simulink model "jerkControl2017"  (Simulink 8.9)
settings: Solver=FixedStepDiscrete  StartTime=0.0  StopTime="Config.SIMULATION_TIME "  FixedStep=Config.Ts  RelTol=1e-3  EnableMultiTasking=on
InitFcn:
  | %% initialize the simulation
  | cd(fileparts(which(bdroot)));
  | initJerkControl;
StopFcn:
  | %% stop the simulation
  | cd(fileparts(which(bdroot)));
  | stopJerkControl;
undefined symbols (not defined in the file or in its folder): Config, DiscIntNeverNeededParam, Gain, Reg, ROBOT_DOF, Sat, Sm
libraries: WBToolboxLibrary x69, simulink x4
(part 1 of 2)
settings Model: Creator=daniele  LastModifiedBy=gnava
settings DataIOCC: SignalLoggingSaveFormat=Dataset
settings OptimizationCC: ExpressionDepthLimit=2147483647  ZeroExternalMemoryAtStartup=off
settings DebuggingCC: SolverPrmCheckMsg=warning  AllowSymbolicDim=off
settings SFSimCC: SimParseCustomCode=off
settings RTWCC: GenCodeOnly=on  TargetLang=C++
settings GRTTargetCC: TargetLangStandard=C++03 (ISO)  CombineOutputUpdateFcns=on  MatFileLogging=off  CodeInterfacePackaging=C++ class  SupportNonFinite=off  GRTInterface=off
settings CPPComponent: GenerateDestructor=on  GenerateExternalIOAccessMethods=None  ParameterMemberVisibility=private  InternalMemberVisibility=private  GenerateParameterAccessMethods=None  GenerateInternalMemberAccessMethods=None  UseOperatorNewForModelRefRegistration=off

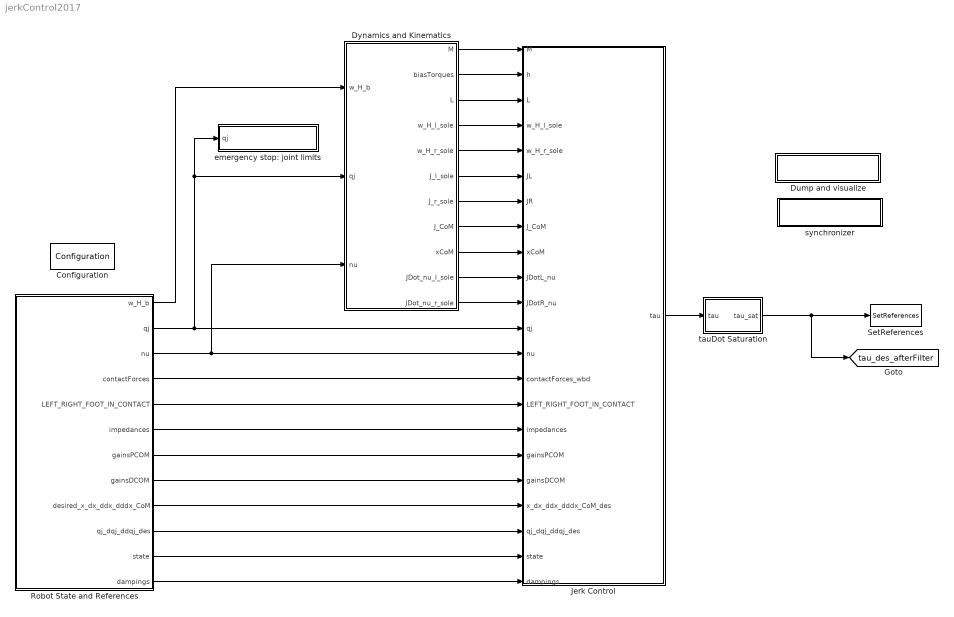
== system jerkControl2017 ==
  Configuration : WBToolboxLibrary/Utilities/Configuration  ConfigSource=Workspace  ConfigObject='WBTConfigRobot'  RobotName='icubSim'  UrdfFile='model.urdf'  ControlledJoints={'l_elbow','l_shoulder_pitch','torso_roll'}  ControlBoardsNames={'left_arm','right_arm','torso'}  LocalName='WBT'  GravityVector=[0,0,-9.81]
      settings: SourceProductName=WholeBodyToolbox
  Dump and visualize : Subsystem
      mask Display: disp('VISUALIZER')
  Dynamics and Kinematics : Subsystem
  Jerk Control : Subsystem
  Robot State and References : Subsystem  Priority=-10
  SetReferences : WBToolboxLibrary/Actuators/SetReferences  controlType=Torque  refSpeed=50  refAcceleration=1000000*(pi/180)
      settings: SourceProductName=WholeBodyToolbox
  emergency stop: joint limits : Subsystem
      mask Display: disp('EMERGENCY STOP')
  synchronizer : Subsystem
      mask Display: disp('SYNCHRONIZER')
  tauDot Saturation : Subsystem
  tag scope: tau_des_afterFilter=global
  wires:
  tauDot Saturation/1(tau_sat) -> SetReferences/1, [tau_des_afterFilter]
  Dynamics and Kinematics/1(M) -> Jerk Control/1(M)
  Dynamics and Kinematics/2(biasTorques) -> Jerk Control/2(h)
  Dynamics and Kinematics/3(L) -> Jerk Control/3(L)
  Dynamics and Kinematics/4(w_H_l_sole) -> Jerk Control/4(w_H_l_sole)
  Dynamics and Kinematics/5(w_H_r_sole) -> Jerk Control/5(w_H_r_sole)
  Dynamics and Kinematics/6(J_l_sole) -> Jerk Control/6(JL)
  Dynamics and Kinematics/7(J_r_sole) -> Jerk Control/7(JR)
  Dynamics and Kinematics/8(J_CoM) -> Jerk Control/8(J_CoM)
  Dynamics and Kinematics/9(xCoM) -> Jerk Control/9(xCoM)
  Dynamics and Kinematics/10(JDot_nu_l_sole) -> Jerk Control/10(JDotL_nu)
  Dynamics and Kinematics/11(JDot_nu_r_sole) -> Jerk Control/11(JDotR_nu)
  Robot State and References/1(w_H_b) -> Dynamics and Kinematics/1(w_H_b)
  Robot State and References/2(qj) -> Jerk Control/12(qj), emergency stop: joint limits/1(qj), Dynamics and Kinematics/2(qj)
  Robot State and References/3(nu) -> Jerk Control/13(nu), Dynamics and Kinematics/3(nu)
  Robot State and References/5(LEFT_RIGHT_FOOT_IN_CONTACT) -> Jerk Control/15(LEFT_RIGHT_FOOT_IN_CONTACT)
  Robot State and References/6(impedances) -> Jerk Control/16(impedances)
  Robot State and References/7(gainsPCOM) -> Jerk Control/17(gainsPCOM)
  Robot State and References/8(gainsDCOM) -> Jerk Control/18(gainsDCOM)
  Robot State and References/9(desired_x_dx_ddx_dddx_CoM) -> Jerk Control/19(x_dx_ddx_dddx_CoM_des)
  Robot State and References/10(qj_dqj_ddqj_des) -> Jerk Control/20(qj_dqj_ddqj_des)
  Jerk Control/1("tau ") -> tauDot Saturation/1(tau)
  Robot State and References/4(contactForces) -> Jerk Control/14(contactForces_wbd)
  Robot State and References/11(state) -> Jerk Control/21(state)
  Robot State and References/12(dampings) -> Jerk Control/22(dampings)

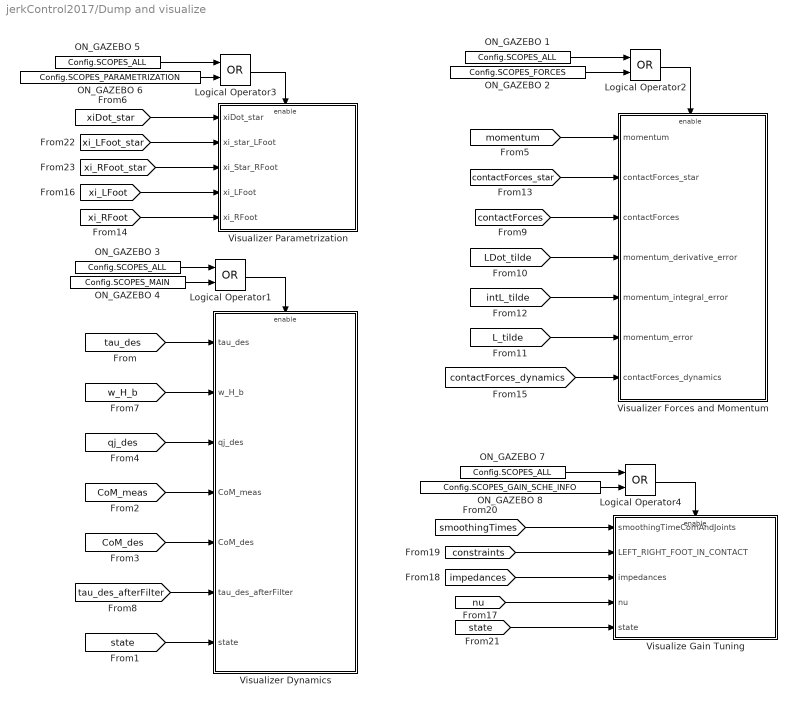
== system jerkControl2017/Dump and visualize ==
  Logical Operator{1..4} (4 alike) : Logic  Operator=OR  AllPortsSameDT=off  OutDataTypeStr=boolean
  ON_GAZEBO {1,3,5,7} (4 alike) : Constant  Value=Config.SCOPES_ALL
  ON_GAZEBO 2 : Constant  Value=Config.SCOPES_FORCES
  ON_GAZEBO 4 : Constant  Value=Config.SCOPES_MAIN
  ON_GAZEBO 6 : Constant  Value=Config.SCOPES_PARAMETRIZATION
  ON_GAZEBO 8 : Constant  Value=Config.SCOPES_GAIN_SCHE_INFO
  "Visualize Gain Tuning  " : Subsystem
  Visualizer Dynamics : Subsystem
  Visualizer Forces and Momentum : Subsystem
  Visualizer Parametrization : Subsystem
  wires:
  ON_GAZEBO 3/1 -> Logical Operator1/1
  ON_GAZEBO 4/1 -> Logical Operator1/2
  Logical Operator1/1 -> Visualizer Dynamics/Enable
  [state] -> Visualizer Dynamics/7(state)
  [CoM_meas] -> Visualizer Dynamics/4(CoM_meas)
  [qj_des] -> Visualizer Dynamics/3(qj_des)
  [w_H_b] -> Visualizer Dynamics/2(w_H_b)
  [tau_des] -> Visualizer Dynamics/1(tau_des)
  [CoM_des] -> Visualizer Dynamics/5(CoM_des)
  [tau_des_afterFilter] -> Visualizer Dynamics/6(tau_des_afterFilter)
  Logical Operator2/1 -> Visualizer Forces and Momentum/Enable
  ON_GAZEBO 2/1 -> Logical Operator2/2
  ON_GAZEBO 1/1 -> Logical Operator2/1
  [momentum] -> Visualizer Forces and Momentum/1(momentum)
  [xiDot_star] -> Visualizer Parametrization/1(xiDot_star)
  ON_GAZEBO 5/1 -> Logical Operator3/1
  Logical Operator3/1 -> Visualizer Parametrization/Enable
  ON_GAZEBO 6/1 -> Logical Operator3/2
  [contactForces_star] -> Visualizer Forces and Momentum/2(contactForces_star)
  [contactForces] -> Visualizer Forces and Momentum/3(contactForces)
  [LDot_tilde] -> Visualizer Forces and Momentum/4(momentum_derivative_error)
  [intL_tilde] -> Visualizer Forces and Momentum/5(momentum_integral_error)
  [L_tilde] -> Visualizer Forces and Momentum/6(momentum_error)
  [contactForces_dynamics] -> Visualizer Forces and Momentum/7(contactForces_dynamics)
  ON_GAZEBO 7/1 -> Logical Operator4/1
  ON_GAZEBO 8/1 -> Logical Operator4/2
  Logical Operator4/1 -> "Visualize Gain Tuning  "/Enable
  [nu] -> "Visualize Gain Tuning  "/4(nu)
  [impedances] -> "Visualize Gain Tuning  "/3(impedances)
  [constraints] -> "Visualize Gain Tuning  "/2(LEFT_RIGHT_FOOT_IN_CONTACT)
  [smoothingTimes] -> "Visualize Gain Tuning  "/1(smoothingTimeComAndJoints)
  [state] -> "Visualize Gain Tuning  "/5(state)
  [xi_LFoot_star] -> Visualizer Parametrization/2(xi_star_LFoot)
  [xi_RFoot] -> Visualizer Parametrization/5(xi_RFoot)
  [xi_LFoot] -> Visualizer Parametrization/4(xi_LFoot)
  [xi_RFoot_star] -> Visualizer Parametrization/3(xi_Star_RFoot)

== system jerkControl2017/Dynamics and Kinematics ==
  w_H_b : Inport
  qj : Inport  Port=2
  nu : Inport  Port=3
  Dynamics : Subsystem
  Kinematics : Subsystem
  M : Outport
  biasTorques : Outport  Port=2
  L : Outport  Port=3
  w_H_l_sole : Outport  Port=4
  w_H_r_sole : Outport  Port=5
  J_l_sole : Outport  Port=6
  J_r_sole : Outport  Port=7
  J_CoM : Outport  Port=8
  xCoM : Outport  Port=9
  JDot_nu_l_sole : Outport  Port=10
  JDot_nu_r_sole : Outport  Port=11
  wires:
  w_H_b/1 -> Kinematics/3(w_H_b), Dynamics/1(w_H_b)
  qj/1 -> Dynamics/2(qj), Kinematics/2(qj)
  nu/1 -> Dynamics/3(nu), Kinematics/1(nu)
  Dynamics/1(M) -> M/1
  Dynamics/2(biasTorques) -> biasTorques/1
  Dynamics/3(L) -> L/1
  Kinematics/7(JDot_nu_l_sole) -> JDot_nu_l_sole/1
  Kinematics/8(JDot_nu_r_sole) -> JDot_nu_r_sole/1
  Kinematics/4(J_r_sole) -> J_r_sole/1
  Kinematics/1(w_H_l_sole) -> w_H_l_sole/1
  Kinematics/3(J_l_sole) -> J_l_sole/1
  Kinematics/5(J_CoM) -> J_CoM/1
  Kinematics/6(xCoM) -> xCoM/1
  Kinematics/2(w_H_r_sole) -> w_H_r_sole/1

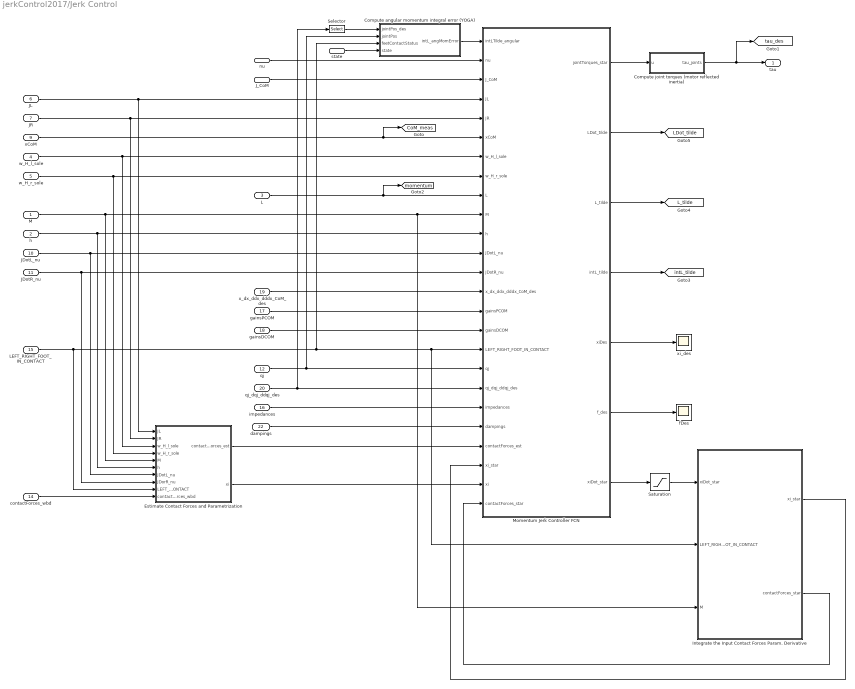
== system jerkControl2017/Jerk Control ==
  M : Inport
  h : Inport  Port=2
  L : Inport  Port=3
  w_H_l_sole : Inport  Port=4
  w_H_r_sole : Inport  Port=5
  JL : Inport  Port=6
  JR : Inport  Port=7
  J_CoM : Inport  Port=8
  xCoM : Inport  Port=9
  JDotL_nu : Inport  Port=10
  JDotR_nu : Inport  Port=11
  qj : Inport  Port=12
  nu : Inport  Port=13
  contactForces_wbd : Inport  Port=14
  LEFT_RIGHT_FOOT_IN_CONTACT : Inport  Port=15
  impedances : Inport  Port=16
  gainsPCOM : Inport  Port=17
  gainsDCOM : Inport  Port=18
  x_dx_ddx_dddx_CoM_des : Inport  Port=19
  qj_dqj_ddqj_des : Inport  Port=20
  state : Inport  Port=21
  dampings : Inport  Port=22
  Compute angular momentum integral error (YOGA) : Subsystem
  Compute joint torques (motor reflected inertia) : Subsystem
  Estimate Contact Forces and Parametrization : Subsystem
  Integrate the Input Contact Forces Param. Derivative : Subsystem
  "Momentum Jerk Controller FCN " : MATLAB Function  TreatAsAtomicUnit=on
  Saturation : Saturate  UpperLimit=Sat.xiDot  LowerLimit=-Sat.xiDot
  Selector : Selector  NumberOfDimensions=2  InputPortWidth=3  IndexOptions=Index vector (dialog),Index vector (dialog)  Indices=[1:ROBOT_DOF],1  OutputSizes=1,1
  fDes : Scope
  xi_des : Scope
  "tau " : Outport
  tag scope: CoM_meas=global, LDot_tilde=global, L_tilde=global, intL_tilde=global, momentum=global, tau_des=global
  wires:
  w_H_l_sole/1 -> Estimate Contact Forces and Parametrization/3(w_H_l_sole), "Momentum Jerk Controller FCN "/7(w_H_l_sole)
  w_H_r_sole/1 -> "Momentum Jerk Controller FCN "/8(w_H_r_sole), Estimate Contact Forces and Parametrization/4(w_H_r_sole)
  x_dx_ddx_dddx_CoM_des/1 -> "Momentum Jerk Controller FCN "/14(x_dx_ddx_dddx_CoM_des)
  nu/1 -> "Momentum Jerk Controller FCN "/2(nu)
  gainsPCOM/1 -> "Momentum Jerk Controller FCN "/15(gainsPCOM)
  Compute angular momentum integral error (YOGA)/1(intL_angMomError) -> "Momentum Jerk Controller FCN "/1(intLTilde_angular)
  qj_dqj_ddqj_des/1 -> "Momentum Jerk Controller FCN "/19(qj_dqj_ddqj_des), Selector/1
  gainsDCOM/1 -> "Momentum Jerk Controller FCN "/16(gainsDCOM)
  impedances/1 -> "Momentum Jerk Controller FCN "/20(impedances)
  xCoM/1 -> "Momentum Jerk Controller FCN "/6(xCoM), [CoM_meas]
  qj/1 -> "Momentum Jerk Controller FCN "/18(qj), Compute angular momentum integral error (YOGA)/2(jointPos)
  Selector/1 -> Compute angular momentum integral error (YOGA)/1(jointPos_des)
  J_CoM/1 -> "Momentum Jerk Controller FCN "/3(J_CoM)
  "Momentum Jerk Controller FCN "/7(xiDot_star) -> Saturation/1
  h/1 -> "Momentum Jerk Controller FCN "/11(h), Estimate Contact Forces and Parametrization/6(h)
  JR/1 -> "Momentum Jerk Controller FCN "/5(JR), Estimate Contact Forces and Parametrization/2(JR)
  L/1 -> [momentum], "Momentum Jerk Controller FCN "/9(L)
  state/1 -> Compute angular momentum integral error (YOGA)/4(state)
  LEFT_RIGHT_FOOT_IN_CONTACT/1 -> Integrate the Input Contact Forces Param. Derivative/2(LEFT_RIGHT_FOOT_IN_CONTACT), "Momentum Jerk Controller FCN "/17(LEFT_RIGHT_FOOT_IN_CONTACT), Compute angular momentum integral error (YOGA)/3(feetContactStatus), Estimate Contact Forces and Parametrization/9(LEFT_RIGHT_FOOT_IN_CONTACT)
  JDotR_nu/1 -> "Momentum Jerk Controller FCN "/13(JDotR_nu), Estimate Contact Forces and Parametrization/8(JDorR_nu)
  Integrate the Input Contact Forces Param. Derivative/1(xi_star) -> "Momentum Jerk Controller FCN "/23(xi_star)
  Integrate the Input Contact Forces Param. Derivative/2(contactForces_star) -> "Momentum Jerk Controller FCN "/25(contactForces_star)
  "Momentum Jerk Controller FCN "/4(intL_tilde) -> [intL_tilde]
  "Momentum Jerk Controller FCN "/3(L_tilde) -> [L_tilde]
  "Momentum Jerk Controller FCN "/2(LDot_tilde) -> [LDot_tilde]
  dampings/1 -> "Momentum Jerk Controller FCN "/21(dampings)
  Saturation/1 -> Integrate the Input Contact Forces Param. Derivative/1(xiDot_star)
  contactForces_wbd/1 -> Estimate Contact Forces and Parametrization/10(contactForces_wbd)
  JL/1 -> "Momentum Jerk Controller FCN "/4(JL), Estimate Contact Forces and Parametrization/1(JL)
  JDotL_nu/1 -> "Momentum Jerk Controller FCN "/12(JDotL_nu), Estimate Contact Forces and Parametrization/7(JDotL_nu)
  Estimate Contact Forces and Parametrization/1(contactForces_est) -> "Momentum Jerk Controller FCN "/22(contactForces_est)
  "Momentum Jerk Controller FCN "/1(jointTorques_star) -> Compute joint torques (motor reflected inertia)/1(u)
  Compute joint torques (motor reflected inertia)/1(tau_joints) -> [tau_des], "tau "/1
  M/1 -> Integrate the Input Contact Forces Param. Derivative/3(M), "Momentum Jerk Controller FCN "/10(M), Estimate Contact Forces and Parametrization/5(M)
  Estimate Contact Forces and Parametrization/2(xi) -> "Momentum Jerk Controller FCN "/24(xi)
  "Momentum Jerk Controller FCN "/5(xiDes) -> xi_des/1
  "Momentum Jerk Controller FCN "/6(f_des) -> fDes/1

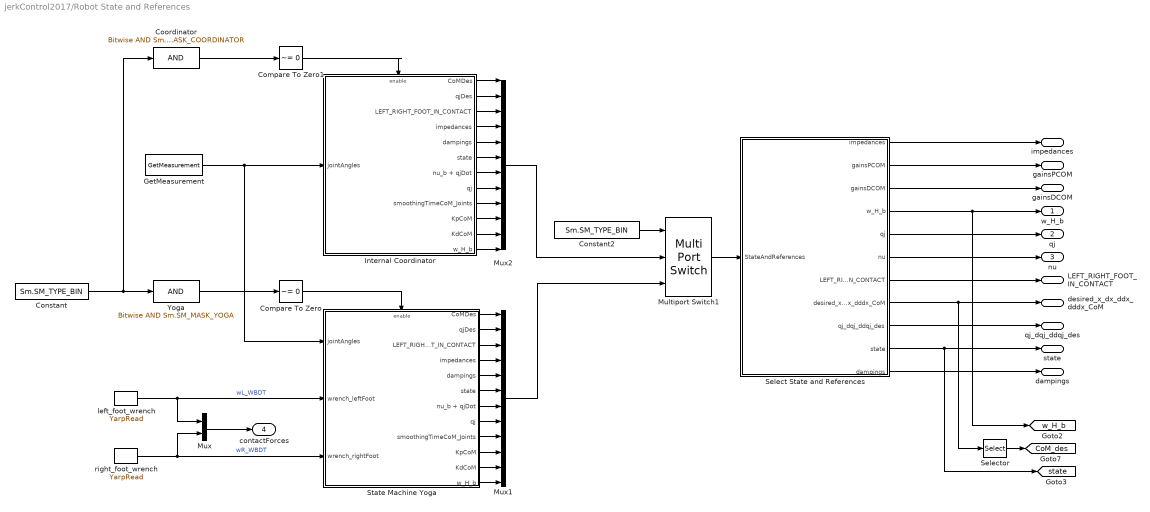
== system jerkControl2017/Robot State and References ==
  Compare To Zero : simulink/Logic and Bit Operations/Compare To Zero  relop=~=  OutDataTypeStr=boolean
  Compare To Zero1 : simulink/Logic and Bit Operations/Compare To Zero  relop=~=  OutDataTypeStr=boolean
  Constant : Constant  Priority=-10  Value=Sm.SM_TYPE_BIN  OutDataTypeStr=uint8
  Constant2 : Constant  Priority=-10  Value=Sm.SM_TYPE_BIN  OutDataTypeStr=uint8
  Coordinator : simulink/Logic and Bit Operations/Bitwise Operator  logicop=AND  UseBitMask=on  BitMask=Sm.SM_MASK_COORDINATOR  BitMaskRealWorld=Stored Integer
  GetMeasurement : WBToolboxLibrary/States/GetMeasurement  measuredType=Joints Position
      settings: SourceProductName=WholeBodyToolbox
  Internal Coordinator : Subsystem
  Multiport Switch1 : MultiPortSwitch  DataPortOrder=Specify indices  DataPortIndices={1, 2}
  Mux : Mux  Inputs=2
  Mux1 : Mux  Inputs=12
  Mux2 : Mux  Inputs=12
  Select State and References : Subsystem
  Selector : Selector  NumberOfDimensions=2  InputPortWidth=3  IndexOptions=Index vector (dialog),Index vector (dialog)  Indices=[1 2 3],[1]  OutputSizes=1,1
  State Machine Yoga : Subsystem  Priority=-100
  Yoga : simulink/Logic and Bit Operations/Bitwise Operator  logicop=AND  UseBitMask=on  BitMask=Sm.SM_MASK_YOGA  BitMaskRealWorld=Stored Integer
  left_foot_wrench : WBToolboxLibrary/Utilities/YarpRead  portName=Ports.WRENCH_LEFT_FOOT  signalSize=6  timeout=0.5  blocking=off  timestamp=off  autoconnect=on  errorOnConnection=on
      settings: SourceProductName=WholeBodyToolbox
  right_foot_wrench : WBToolboxLibrary/Utilities/YarpRead  portName=Ports.WRENCH_RIGHT_FOOT  signalSize=6  timeout=0.5  blocking=off  timestamp=off  autoconnect=on  errorOnConnection=on
      settings: SourceProductName=WholeBodyToolbox
  w_H_b : Outport
  qj : Outport  Port=2
  nu : Outport  Port=3
  contactForces : Outport  Port=4
  LEFT_RIGHT_FOOT_IN_CONTACT : Outport  Port=5
  impedances : Outport  Port=6
  gainsPCOM : Outport  Port=7
  gainsDCOM : Outport  Port=8
  desired_x_dx_ddx_dddx_CoM : Outport  Port=9
  qj_dqj_ddqj_des : Outport  Port=10
  state : Outport  Port=11
  dampings : Outport  Port=12
  tag scope: CoM_des=global, state=global, w_H_b=global
  wires:
  Constant/1 -> Coordinator/1, Yoga/1
  State Machine Yoga/3(LEFT_RIGHT_FOOT_IN_CONTACT) -> Mux1/3
  State Machine Yoga/2(qjDes) -> Mux1/2
  State Machine Yoga/1(CoMDes) -> Mux1/1
  Internal Coordinator/1(CoMDes) -> Mux2/1
  Internal Coordinator/2(qjDes) -> Mux2/2
  Internal Coordinator/3(LEFT_RIGHT_FOOT_IN_CONTACT) -> Mux2/3
  State Machine Yoga/4(impedances) -> Mux1/4
  Internal Coordinator/4(impedances) -> Mux2/4
  State Machine Yoga/6(state) -> Mux1/6
  Internal Coordinator/6(state) -> Mux2/6
  Internal Coordinator/7(nu_b + qjDot) -> Mux2/7
  Internal Coordinator/8(qj) -> Mux2/8
  State Machine Yoga/7(nu_b + qjDot) -> Mux1/7
  State Machine Yoga/8(qj) -> Mux1/8
  Coordinator/1 -> Compare To Zero1/1
  Yoga/1 -> Compare To Zero/1
  Compare To Zero/1 -> State Machine Yoga/Enable
  Compare To Zero1/1 -> Internal Coordinator/Enable
  Internal Coordinator/9(smoothingTimeCoM_Joints) -> Mux2/9
  State Machine Yoga/9(smoothingTimeCoM_Joints) -> Mux1/9
  State Machine Yoga/10(KpCoM) -> Mux1/10
  State Machine Yoga/11(KdCoM) -> Mux1/11
  Internal Coordinator/10(KpCoM) -> Mux2/10
  Internal Coordinator/11(KdCoM) -> Mux2/11
  Constant2/1 -> Multiport Switch1/1
  GetMeasurement/1 -> Internal Coordinator/1(jointAngles), State Machine Yoga/1(jointAngles)
  State Machine Yoga/12(w_H_b) -> Mux1/12
  Internal Coordinator/12(w_H_b) -> Mux2/12
  Mux2/1 -> Multiport Switch1/2
  Mux1/1 -> Multiport Switch1/3
  Multiport Switch1/1 -> Select State and References/1(StateAndReferences)
  Select State and References/1(impedances) -> impedances/1
  Select State and References/2(gainsPCOM) -> gainsPCOM/1
  Select State and References/3(gainsDCOM) -> gainsDCOM/1
  Select State and References/4(w_H_b) -> w_H_b/1, [w_H_b]
  Select State and References/5(qj) -> qj/1
  Select State and References/6(nu) -> nu/1
  Select State and References/7(LEFT_RIGHT_FOOT_IN_CONTACT) -> LEFT_RIGHT_FOOT_IN_CONTACT/1
  Select State and References/8(desired_x_dx_ddx_dddx_CoM) -> desired_x_dx_ddx_dddx_CoM/1, Selector/1
  Select State and References/9(qj_dqj_ddqj_des) -> qj_dqj_ddqj_des/1
  Select State and References/10(state) -> state/1, [state]
  Selector/1 -> [CoM_des]
  left_foot_wrench/1 -> Mux/1, State Machine Yoga/2(wrench_leftFoot)  "wL_WBDT"
  right_foot_wrench/1 -> Mux/2, State Machine Yoga/3(wrench_rightFoot)  "wR_WBDT"
  Mux/1 -> contactForces/1
  State Machine Yoga/5(dampings) -> Mux1/5
  Internal Coordinator/5(dampings) -> Mux2/5
  Select State and References/11(dampings) -> dampings/1

== system jerkControl2017/emergency stop: joint limits ==
  qj : Inport
  ON_GAZEBO 1 : Constant  Value=Config.EMERGENCY_STOP_WITH_JOINTS_LIMITS
  ON_GAZEBO 2 : Constant  Value=Config.EMERGENCY_STOP_WITH_ENCODER_SPIKES
  STOP IF JOINTS HIT THE LIMITS : Subsystem
  STOP IF THERE ARE SPIKES IN THE ENCODERS : Subsystem
  wires:
  ON_GAZEBO 1/1 -> STOP IF JOINTS HIT THE LIMITS/Enable
  qj/1 -> STOP IF THERE ARE SPIKES IN THE ENCODERS/1(qj), STOP IF JOINTS HIT THE LIMITS/1(qj)
  ON_GAZEBO 2/1 -> STOP IF THERE ARE SPIKES IN THE ENCODERS/Enable

== system jerkControl2017/synchronizer ==
  GAZEBO_SYNCHRONIZER : Subsystem
  Logical Operator : Logic  Operator=NOT  AllPortsSameDT=off  OutDataTypeStr=boolean
  "ON_GAZEBO " : Constant  Value=Config.ON_GAZEBO
  REAL_TIME_SYNC : Subsystem
  To Workspace : ToWorkspace  VariableName=yarp_time  SaveFormat=Structure With Time  SampleTime=-1
  Yarp Clock : WBToolboxLibrary/Utilities/Yarp Clock
      settings: SourceProductName=WholeBodyToolbox
  wires:
  Logical Operator/1 -> REAL_TIME_SYNC/Enable
  "ON_GAZEBO "/1 -> GAZEBO_SYNCHRONIZER/Enable, Logical Operator/1
  Yarp Clock/1 -> To Workspace/1

== system jerkControl2017/tauDot Saturation ==
  tau : Inport
  Constant : Constant  Value=Config.SATURATE_TORQUE_DERIVATIVE
  Constant1 : Constant  Value=Config.Ts
  Constant2 : Constant  Value=Sat.uDotMax
  Saturate Torque Derivative : MATLAB Function  TreatAsAtomicUnit=on
  Saturation : Saturate  UpperLimit=Sat.torque  LowerLimit=-Sat.torque
  Switch : Switch  Criteria=u2 > Threshold
  "holder " : WBToolboxLibrary/Utilities/holder 
      settings: SourceProductName=WholeBodyToolbox
  tau_sat : Outport
  wires:
  Switch/1 -> Saturation/1
  Constant/1 -> Switch/2
  Constant1/1 -> Saturate Torque Derivative/3(tStep)
  Saturate Torque Derivative/1(uSat) -> Switch/1
  "holder "/1 -> Saturate Torque Derivative/2(u_0)
  Saturation/1 -> tau_sat/1
  tau/1 -> Switch/3, Saturate Torque Derivative/1(u), "holder "/1
  Constant2/1 -> Saturate Torque Derivative/4(uDotMax)

== system jerkControl2017/Dump and visualize/Visualize Gain Tuning   ==
  smoothingTimeComAndJoints : Inport
  LEFT_RIGHT_FOOT_IN_CONTACT : Inport  Port=2
  impedances : Inport  Port=3
  nu : Inport  Port=4
  state : Inport  Port=5
  Enable : EnablePort
  Demux : Demux  Outputs=2
  Demux1 : Demux  Outputs=Config.numOfJointsForEachControlboard
  Demux2 : Demux  Outputs=Config.numOfJointsForEachControlboard
  Gain : Gain  Gain=180/pi
  Gain1 : Gain  Gain=180/pi
  Impedances : Scope  NumInputPorts=6
  Left right foot in contact : Scope
  Selector1 : Selector  InputPortWidth=6+ROBOT_DOF  IndexOptions=Index vector (dialog)  Indices=[7:6+ROBOT_DOF]  OutputSizes=1
  Selector2 : Selector  InputPortWidth=6+ROBOT_DOF  IndexOptions=Index vector (dialog)  Indices=[1:6]  OutputSizes=1
  "joint velocities " : Scope  NumInputPorts=6
  jointsSmoothingTime : Scope  NumInputPorts=2
  linear and angular  base velocity : Scope  NumInputPorts=3
  wires:
  state/1 -> "joint velocities "/6, linear and angular  base velocity/3, Impedances/6, jointsSmoothingTime/2  "state"
  LEFT_RIGHT_FOOT_IN_CONTACT/1 -> Left right foot in contact/1
  impedances/1 -> Demux1/1
  smoothingTimeComAndJoints/1 -> jointsSmoothingTime/1  "smoothingTimeComAndJoints"
  Demux1/4 -> Impedances/4  "left_leg"
  Demux1/5 -> Impedances/5  "right_leg"
  Demux1/3 -> Impedances/3  "right_arm"
  Demux1/1 -> Impedances/1  "torso"
  Demux1/2 -> Impedances/2  "left_arm"
  Selector1/1 -> Gain/1
  Demux2/4 -> "joint velocities "/4  "left_leg"
  Demux2/3 -> "joint velocities "/3  "right_arm"
  Demux2/1 -> "joint velocities "/1  "torso"
  Demux2/2 -> "joint velocities "/2  "left_arm"
  nu/1 -> Selector1/1, Selector2/1
  Selector2/1 -> Demux/1
  Demux/1 -> linear and angular  base velocity/1
  Demux/2 -> Gain1/1
  Gain/1 -> Demux2/1
  Gain1/1 -> linear and angular  base velocity/2
  Demux2/5 -> "joint velocities "/5  "right_leg"

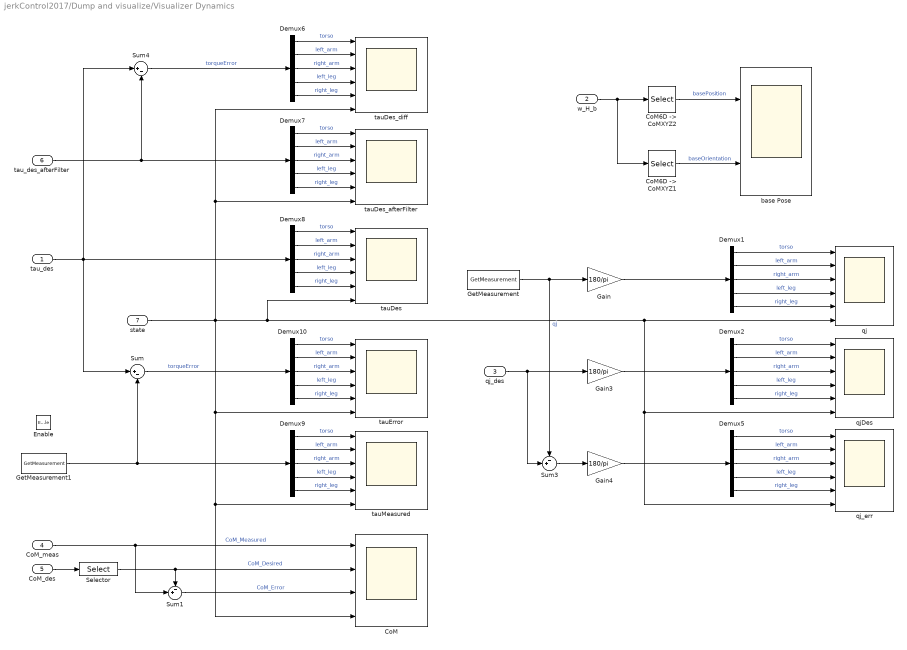
== system jerkControl2017/Dump and visualize/Visualizer Dynamics ==
  tau_des : Inport
  w_H_b : Inport  Port=2
  qj_des : Inport  Port=3
  CoM_meas : Inport  Port=4
  CoM_des : Inport  Port=5
  tau_des_afterFilter : Inport  Port=6
  state : Inport  Port=7
  Enable : EnablePort
  CoM : Scope  NumInputPorts=4
  "CoM6D ->  CoMXYZ1" : Selector  NumberOfDimensions=2  InputPortWidth=7  IndexOptions=Index vector (dialog),Index vector (dialog)  Indices=[1 2 3],[1 2 3]  OutputSizes=1,1
  "CoM6D ->  CoMXYZ2" : Selector  NumberOfDimensions=2  InputPortWidth=7  IndexOptions=Index vector (dialog),Index vector (dialog)  Indices=[1 2 3],[4]  OutputSizes=1,1
  Demux{1..2,5..10} (8 alike) : Demux  Outputs=Config.numOfJointsForEachControlboard
  Gain : Gain  Gain=180/pi
  Gain3 : Gain  Gain=180/pi
  Gain4 : Gain  Gain=180/pi
  GetMeasurement : WBToolboxLibrary/States/GetMeasurement  measuredType=Joints Position
      settings: SourceProductName=WholeBodyToolbox
  GetMeasurement1 : WBToolboxLibrary/States/GetMeasurement  measuredType=Joints Torque
      settings: SourceProductName=WholeBodyToolbox
  Selector : Selector  NumberOfDimensions=2  IndexOptions=Index vector (dialog),Index vector (dialog)  Indices=[1:3],1  OutputSizes=1,1
  Sum : Sum  Inputs=|+-
  Sum1 : Sum  Inputs=-+|
  Sum3 : Sum  Inputs=-+|
  Sum4 : Sum  Inputs=|+-
  base Pose : Scope  NumInputPorts=2
  qj : Scope  NumInputPorts=6
  qjDes : Scope  NumInputPorts=6
  qj_err : Scope  NumInputPorts=6
  tauDes : Scope  NumInputPorts=6
  tauDes_afterFilter : Scope  NumInputPorts=6
  tauDes_diff : Scope  NumInputPorts=6
  tauError : Scope  NumInputPorts=6
  tauMeasured : Scope  NumInputPorts=6
  wires:
  CoM_meas/1 -> Sum1/2, CoM/1  "CoM_Measured"
  CoM_des/1 -> Selector/1
  Gain/1 -> Demux1/1
  GetMeasurement/1 -> Gain/1, Sum3/1  "qj"
  Demux1/5 -> qj/5  "right_leg"
  Demux1/1 -> qj/1  "torso"
  Demux1/2 -> qj/2  "left_arm"
  Demux1/4 -> qj/4  "left_leg"
  Demux1/3 -> qj/3  "right_arm"
  GetMeasurement1/1 -> Demux9/1, Sum/2
  Demux8/5 -> tauDes/5  "right_leg"
  Demux8/1 -> tauDes/1  "torso"
  Demux8/2 -> tauDes/2  "left_arm"
  Demux8/4 -> tauDes/4  "left_leg"
  Demux8/3 -> tauDes/3  "right_arm"
  Demux10/5 -> tauError/5  "right_leg"
  Demux10/1 -> tauError/1  "torso"
  Demux10/2 -> tauError/2  "left_arm"
  Demux10/4 -> tauError/4  "left_leg"
  Demux10/3 -> tauError/3  "right_arm"
  Sum/1 -> Demux10/1  "torqueError"
  Demux9/5 -> tauMeasured/5  "right_leg"
  Demux9/1 -> tauMeasured/1  "torso"
  Demux9/2 -> tauMeasured/2  "left_arm"
  Demux9/4 -> tauMeasured/4  "left_leg"
  Demux9/3 -> tauMeasured/3  "right_arm"
  qj_des/1 -> Sum3/2, Gain3/1
  Gain3/1 -> Demux2/1
  Demux2/5 -> qjDes/5  "right_leg"
  Demux2/1 -> qjDes/1  "torso"
  Demux2/2 -> qjDes/2  "left_arm"
  Demux2/4 -> qjDes/4  "left_leg"
  Demux2/3 -> qjDes/3  "right_arm"
  Gain4/1 -> Demux5/1
  Demux5/5 -> qj_err/5  "right_leg"
  Demux5/1 -> qj_err/1  "torso"
  Demux5/2 -> qj_err/2  "left_arm"
  Demux5/4 -> qj_err/4  "left_leg"
  Demux5/3 -> qj_err/3  "right_arm"
  Sum3/1 -> Gain4/1
  Selector/1 -> Sum1/1, CoM/2  "CoM_Desired"
  w_H_b/1 -> "CoM6D ->  CoMXYZ1"/1, "CoM6D ->  CoMXYZ2"/1
  "CoM6D ->  CoMXYZ2"/1 -> base Pose/1  "basePosition"
  "CoM6D ->  CoMXYZ1"/1 -> base Pose/2  "baseOrientation"
  Demux7/4 -> tauDes_afterFilter/4  "left_leg"
  Demux7/5 -> tauDes_afterFilter/5  "right_leg"
  Demux7/2 -> tauDes_afterFilter/2  "left_arm"
  Demux7/1 -> tauDes_afterFilter/1  "torso"
  Demux7/3 -> tauDes_afterFilter/3  "right_arm"
  tau_des_afterFilter/1 -> Demux7/1, Sum4/2
  Sum4/1 -> Demux6/1  "torqueError"
  tau_des/1 -> Demux8/1, Sum/1, Sum4/1
  Demux6/5 -> tauDes_diff/5  "right_leg"
  state/1 -> tauDes_diff/6, tauDes_afterFilter/6, qj_err/6, qjDes/6, qj/6, tauDes/6, CoM/4, tauMeasured/6, tauError/6
  Demux6/3 -> tauDes_diff/3  "right_arm"
  Demux6/2 -> tauDes_diff/2  "left_arm"
  Demux6/4 -> tauDes_diff/4  "left_leg"
  Demux6/1 -> tauDes_diff/1  "torso"
  Sum1/1 -> CoM/3  "CoM_Error"

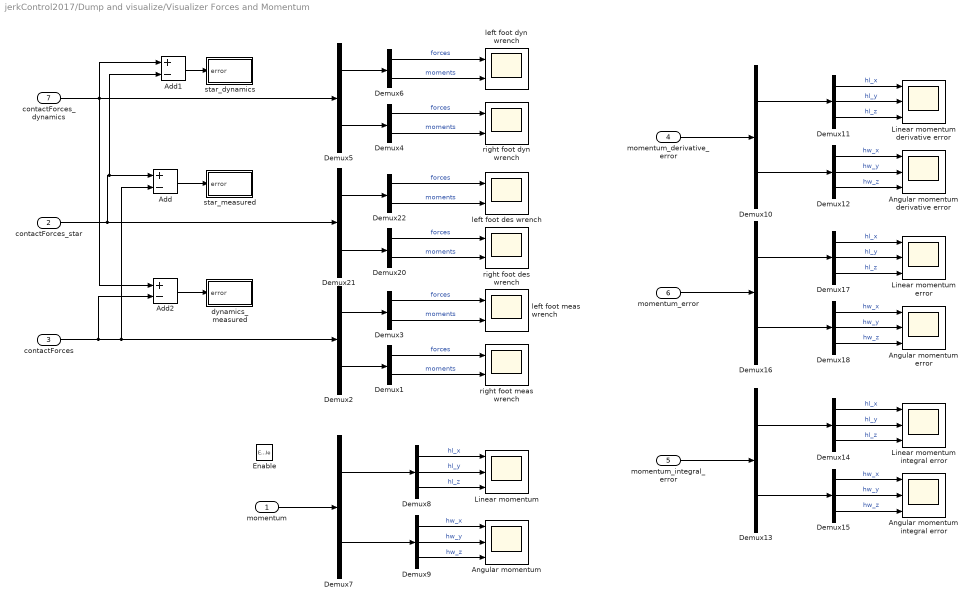
== system jerkControl2017/Dump and visualize/Visualizer Forces and Momentum ==
  momentum : Inport
  contactForces_star : Inport  Port=2
  contactForces : Inport  Port=3
  momentum_derivative_error : Inport  Port=4
  momentum_integral_error : Inport  Port=5
  momentum_error : Inport  Port=6
  contactForces_dynamics : Inport  Port=7
  Enable : EnablePort
  Add : Sum  Inputs=+-
  Add1 : Sum  Inputs=+-
  Add2 : Sum  Inputs=+-
  Angular momentum : Scope  NumInputPorts=3
  Angular momentum derivative error : Scope  NumInputPorts=3
  Angular momentum error : Scope  NumInputPorts=3
  Angular momentum integral error : Scope  NumInputPorts=3
  Demux{1,3..4,6,20,22} (6 alike) : Demux  Outputs=[3;3]
  Demux{7,10,13,16} (4 alike) : Demux  Outputs=2
  Demux{8..9,11..12,14..15,17..18} (8 alike) : Demux  Outputs=3
  Demux2 : Demux  Outputs=[6;6]
  Demux21 : Demux  Outputs=[6;6]
  Demux5 : Demux  Outputs=[6;6]
  Linear momentum : Scope  NumInputPorts=3
  Linear momentum derivative error : Scope  NumInputPorts=3
  Linear momentum error : Scope  NumInputPorts=3
  Linear momentum integral error : Scope  NumInputPorts=3
  dynamics_measured : Subsystem
  left foot des wrench : Scope  NumInputPorts=2
  left foot dyn wrench : Scope  NumInputPorts=2
  left foot meas wrench : Scope  NumInputPorts=2
  right foot des wrench : Scope  NumInputPorts=2
  right foot dyn wrench : Scope  NumInputPorts=2
  right foot meas wrench : Scope  NumInputPorts=2
  star_dynamics : Subsystem
  star_measured : Subsystem
  wires:
  Demux9/3 -> Angular momentum/3  "hw_z"
  Demux8/1 -> Linear momentum/1  "hl_x"
  Demux8/2 -> Linear momentum/2  "hl_y"
  Demux7/2 -> Demux9/1
  Demux9/2 -> Angular momentum/2  "hw_y"
  Demux7/1 -> Demux8/1
  momentum/1 -> Demux7/1
  Demux8/3 -> Linear momentum/3  "hl_z"
  Demux9/1 -> Angular momentum/1  "hw_x"
  Demux11/1 -> Linear momentum derivative error/1  "hl_x"
  momentum_derivative_error/1 -> Demux10/1
  Demux10/1 -> Demux11/1
  Demux12/1 -> Angular momentum derivative error/1  "hw_x"
  Demux12/2 -> Angular momentum derivative error/2  "hw_y"
  Demux11/2 -> Linear momentum derivative error/2  "hl_y"
  Demux11/3 -> Linear momentum derivative error/3  "hl_z"
  Demux10/2 -> Demux12/1
  Demux12/3 -> Angular momentum derivative error/3  "hw_z"
  Demux14/1 -> Linear momentum integral error/1  "hl_x"
  momentum_integral_error/1 -> Demux13/1
  Demux13/1 -> Demux14/1
  Demux15/1 -> Angular momentum integral error/1  "hw_x"
  Demux15/2 -> Angular momentum integral error/2  "hw_y"
  Demux14/2 -> Linear momentum integral error/2  "hl_y"
  Demux14/3 -> Linear momentum integral error/3  "hl_z"
  Demux13/2 -> Demux15/1
  Demux15/3 -> Angular momentum integral error/3  "hw_z"
  Demux17/1 -> Linear momentum error/1  "hl_x"
  momentum_error/1 -> Demux16/1
  Demux16/1 -> Demux17/1
  Demux18/1 -> Angular momentum error/1  "hw_x"
  Demux18/2 -> Angular momentum error/2  "hw_y"
  Demux17/2 -> Linear momentum error/2  "hl_y"
  Demux17/3 -> Linear momentum error/3  "hl_z"
  Demux16/2 -> Demux18/1
  Demux18/3 -> Angular momentum error/3  "hw_z"
  Demux20/2 -> right foot des wrench/2  "moments"
  Demux21/2 -> Demux20/1
  Demux21/1 -> Demux22/1
  Demux22/2 -> left foot des wrench/2  "moments"
  Demux22/1 -> left foot des wrench/1  "forces"
  Demux20/1 -> right foot des wrench/1  "forces"
  Demux3/2 -> left foot meas wrench/2  "moments"
  Demux3/1 -> left foot meas wrench/1  "forces"
  Demux1/2 -> right foot meas wrench/2  "moments"
  Demux1/1 -> right foot meas wrench/1  "forces"
  Demux2/1 -> Demux3/1
  Demux2/2 -> Demux1/1
  Demux4/2 -> right foot dyn wrench/2  "moments"
  Demux6/2 -> left foot dyn wrench/2  "moments"
  Demux6/1 -> left foot dyn wrench/1  "forces"
  Demux5/2 -> Demux4/1
  Demux4/1 -> right foot dyn wrench/1  "forces"
  Demux5/1 -> Demux6/1
  Add/1 -> star_measured/1(error)
  contactForces_star/1 -> Add1/2, Add/1, Demux21/1
  Add1/1 -> star_dynamics/1(error)
  contactForces_dynamics/1 -> Add2/1, Demux5/1, Add1/1
  contactForces/1 -> Add2/2, Add/2, Demux2/1
  Add2/1 -> dynamics_measured/1(error)

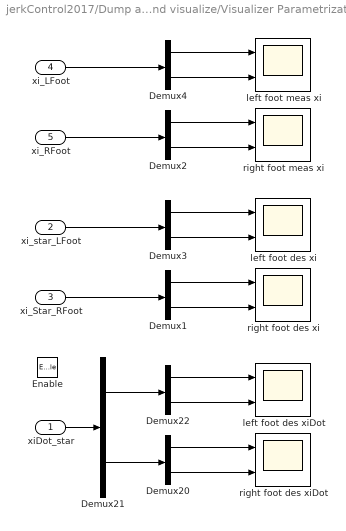
== system jerkControl2017/Dump and visualize/Visualizer Parametrization ==
  xiDot_star : Inport
  xi_star_LFoot : Inport  Port=2
  xi_Star_RFoot : Inport  Port=3
  xi_LFoot : Inport  Port=4
  xi_RFoot : Inport  Port=5
  Enable : EnablePort
  Demux{1..4,20,22} (6 alike) : Demux  Outputs=[3;3]
  Demux21 : Demux  Outputs=[6;6]
  left foot des xi : Scope  NumInputPorts=2
  left foot des xiDot : Scope  NumInputPorts=2
  left foot meas xi : Scope  NumInputPorts=2
  right foot des xi : Scope  NumInputPorts=2
  right foot des xiDot : Scope  NumInputPorts=2
  right foot meas xi : Scope  NumInputPorts=2
  wires:
  Demux20/1 -> right foot des xiDot/1
  Demux21/1 -> Demux22/1
  Demux22/2 -> left foot des xiDot/2
  Demux21/2 -> Demux20/1
  xiDot_star/1 -> Demux21/1
  Demux22/1 -> left foot des xiDot/1
  Demux20/2 -> right foot des xiDot/2
  Demux3/2 -> left foot des xi/2
  xi_star_LFoot/1 -> Demux3/1
  Demux3/1 -> left foot des xi/1
  xi_Star_RFoot/1 -> Demux1/1
  Demux1/1 -> right foot des xi/1
  Demux1/2 -> right foot des xi/2
  Demux2/2 -> right foot meas xi/2
  Demux4/2 -> left foot meas xi/2
  xi_RFoot/1 -> Demux2/1
  Demux2/1 -> right foot meas xi/1
  xi_LFoot/1 -> Demux4/1
  Demux4/1 -> left foot meas xi/1

== system jerkControl2017/Dynamics and Kinematics/Dynamics ==
  w_H_b : Inport
  qj : Inport  Port=2
  nu : Inport  Port=3
  Add motors reflected inertia : Subsystem
  CentroidalMomentum : WBToolboxLibrary/Model/Dynamics/CentroidalMomentum
      settings: SourceProductName=WholeBodyToolbox
  "CoM6D ->  CoMXYZ1" : Selector  InputPortWidth=6+ROBOT_DOF  IndexOptions=Index vector (dialog)  Indices=[7:6+ROBOT_DOF]  OutputSizes=1
  "CoM6D ->  CoMXYZ2" : Selector  InputPortWidth=6+ROBOT_DOF  IndexOptions=Index vector (dialog)  Indices=[1 2 3 4 5 6]  OutputSizes=1
  GetBiasForces : WBToolboxLibrary/Model/Dynamics/GetBiasForces
      settings: SourceProductName=WholeBodyToolbox
  MassMatrix : WBToolboxLibrary/Model/Dynamics/MassMatrix
      settings: SourceProductName=WholeBodyToolbox
  M : Outport
  biasTorques : Outport  Port=2
  L : Outport  Port=3
  wires:
  CentroidalMomentum/1 -> L/1
  GetBiasForces/1 -> biasTorques/1
  w_H_b/1 -> CentroidalMomentum/1, GetBiasForces/1, MassMatrix/1
  qj/1 -> CentroidalMomentum/2, GetBiasForces/2, MassMatrix/2
  "CoM6D ->  CoMXYZ1"/1 -> CentroidalMomentum/4, GetBiasForces/4
  nu/1 -> "CoM6D ->  CoMXYZ1"/1, "CoM6D ->  CoMXYZ2"/1
  MassMatrix/1 -> Add motors reflected inertia/1(M)
  Add motors reflected inertia/1(M_with_motor_inertia) -> M/1
  "CoM6D ->  CoMXYZ2"/1 -> CentroidalMomentum/3, GetBiasForces/3

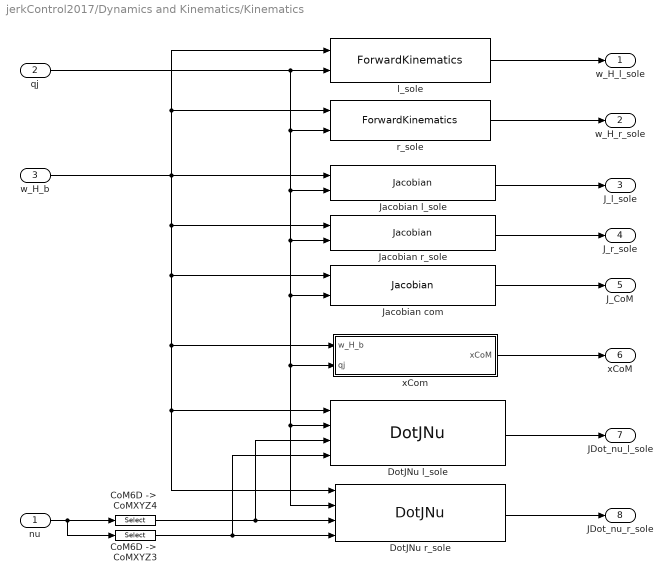
== system jerkControl2017/Dynamics and Kinematics/Kinematics ==
  nu : Inport
  qj : Inport  Port=2
  w_H_b : Inport  Port=3
  "CoM6D ->  CoMXYZ3" : Selector  InputPortWidth=6+ROBOT_DOF  IndexOptions=Index vector (dialog)  Indices=[7:6+ROBOT_DOF]  OutputSizes=1
  "CoM6D ->  CoMXYZ4" : Selector  InputPortWidth=6+ROBOT_DOF  IndexOptions=Index vector (dialog)  Indices=[1 2 3 4 5 6]  OutputSizes=1
  "DotJNu l_sole " : WBToolboxLibrary/Model/Jacobians/DotJNu  frameName=Frames.LEFT_FOOT
      settings: SourceProductName=WholeBodyToolbox
  "DotJNu r_sole   " : WBToolboxLibrary/Model/Jacobians/DotJNu  frameName=Frames.RIGHT_FOOT
      settings: SourceProductName=WholeBodyToolbox
  Jacobian com : WBToolboxLibrary/Model/Jacobians/Jacobian  frameName=Frames.COM
      settings: SourceProductName=WholeBodyToolbox
  Jacobian l_sole : WBToolboxLibrary/Model/Jacobians/Jacobian  frameName=Frames.LEFT_FOOT
      settings: SourceProductName=WholeBodyToolbox
  Jacobian r_sole : WBToolboxLibrary/Model/Jacobians/Jacobian  frameName=Frames.RIGHT_FOOT
      settings: SourceProductName=WholeBodyToolbox
  l_sole : WBToolboxLibrary/Model/Kinematics/ForwardKinematics  frameName=Frames.LEFT_FOOT
      settings: SourceProductName=WholeBodyToolbox
  r_sole : WBToolboxLibrary/Model/Kinematics/ForwardKinematics  frameName=Frames.RIGHT_FOOT
      settings: SourceProductName=WholeBodyToolbox
  xCom : Subsystem
  w_H_l_sole : Outport
  w_H_r_sole : Outport  Port=2
  J_l_sole : Outport  Port=3
  J_r_sole : Outport  Port=4
  J_CoM : Outport  Port=5
  xCoM : Outport  Port=6
  JDot_nu_l_sole : Outport  Port=7
  JDot_nu_r_sole : Outport  Port=8
  wires:
  "CoM6D ->  CoMXYZ3"/1 -> "DotJNu r_sole   "/4, "DotJNu l_sole "/4
  "CoM6D ->  CoMXYZ4"/1 -> "DotJNu r_sole   "/3, "DotJNu l_sole "/3
  nu/1 -> "CoM6D ->  CoMXYZ3"/1, "CoM6D ->  CoMXYZ4"/1
  w_H_b/1 -> Jacobian com/1, "DotJNu l_sole "/1, "DotJNu r_sole   "/1, xCom/1(w_H_b), Jacobian r_sole/1, Jacobian l_sole/1, r_sole/1, l_sole/1
  qj/1 -> Jacobian com/2, xCom/2(qj), "DotJNu r_sole   "/2, "DotJNu l_sole "/2, Jacobian r_sole/2, Jacobian l_sole/2, r_sole/2, l_sole/2
  l_sole/1 -> w_H_l_sole/1
  r_sole/1 -> w_H_r_sole/1
  Jacobian l_sole/1 -> J_l_sole/1
  Jacobian r_sole/1 -> J_r_sole/1
  Jacobian com/1 -> J_CoM/1
  xCom/1(xCoM) -> xCoM/1
  "DotJNu l_sole "/1 -> JDot_nu_l_sole/1
  "DotJNu r_sole   "/1 -> JDot_nu_r_sole/1

== system jerkControl2017/Jerk Control/Compute angular momentum integral error (YOGA) ==
  jointPos_des : Inport
  jointPos : Inport  Port=2
  feetContactStatus : Inport  Port=3
  state : Inport  Port=4
  Add : Sum  Inputs=-+
  CentroidalMomentum : WBToolboxLibrary/Model/Dynamics/CentroidalMomentum
      settings: SourceProductName=WholeBodyToolbox
  Compute base to fixed link transform : Subsystem
  Get Equivalent Base Velocity : MATLAB Function  TreatAsAtomicUnit=on
  Jacobian : WBToolboxLibrary/Model/Jacobians/Jacobian  frameName=Frames.LEFT_FOOT
      settings: SourceProductName=WholeBodyToolbox
  Jacobian1 : WBToolboxLibrary/Model/Jacobians/Jacobian  frameName=Frames.RIGHT_FOOT
      settings: SourceProductName=WholeBodyToolbox
  Select base to world transform : MATLAB Function  TreatAsAtomicUnit=on
  Selector : Selector  InputPortWidth=6  IndexOptions=Index vector (dialog)  Indices=[4 5 6]  OutputSizes=1
  Switch : Switch  Criteria=u2 > Threshold  Threshold=0.1
  intL_angMomError : Outport
  wires:
  jointPos_des/1 -> Add/1, Jacobian1/2, Jacobian/2, CentroidalMomentum/2, Compute base to fixed link transform/1(jointPos)
  jointPos/1 -> Add/2
  Add/1 -> Get Equivalent Base Velocity/4(jointPos_err), CentroidalMomentum/4
  Get Equivalent Base Velocity/1(baseVel_equivalent) -> CentroidalMomentum/3
  CentroidalMomentum/1 -> Selector/1
  Selector/1 -> intL_angMomError/1
  state/1 -> Select base to world transform/1(state)
  Select base to world transform/1(booleanState) -> Switch/2
  Switch/1 -> CentroidalMomentum/1, Jacobian/1, Jacobian1/1
  Compute base to fixed link transform/1(fixed_l_sole_H_b) -> Switch/1
  Compute base to fixed link transform/2(fixed_r_sole_H_b) -> Switch/3
  Jacobian/1 -> Get Equivalent Base Velocity/1(J_l_sole)
  Jacobian1/1 -> Get Equivalent Base Velocity/2(J_r_sole)
  feetContactStatus/1 -> Get Equivalent Base Velocity/3(feetContactStatus)

== system jerkControl2017/Jerk Control/Compute joint torques (motor reflected inertia) ==
  u : Inport
  " 2" : Constant  Value=Config.USE_MOTOR_REFLECTED_INERTIA
  " 3" : Constant  Value=Config.USE_DES_JOINT_ACC_FOR_MOTORS_INERTIA
  "(transpose(T*Gamma))^{-1}*I_m*(T*Gamma)^{-1}1" : MATLAB Function  TreatAsAtomicUnit=on
  Add1 : Sum  Inputs=-+
  Gain1 : Gain  Gain=Config.K_ff
  GetMeasurement1 : WBToolboxLibrary/States/GetMeasurement  measuredType=Joints Acceleration
      settings: SourceProductName=WholeBodyToolbox
  Product1 : Product  Multiplication=Matrix(*)
  Switch2 : Switch  Criteria=u2 > Threshold
  Switch3 : Switch  Criteria=u2 > Threshold
  tau_joints : Outport
  wires:
  " 3"/1 -> Switch3/2
  GetMeasurement1/1 -> Switch3/3
  [qjDDot_des] -> Switch3/1
  " 2"/1 -> Switch2/2
  Switch3/1 -> Product1/2
  Switch2/1 -> tau_joints/1
  Gain1/1 -> Add1/1
  Product1/1 -> Gain1/1
  "(transpose(T*Gamma))^{-1}*I_m*(T*Gamma)^{-1}1"/1(reflectedInertia) -> Product1/1
  u/1 -> Add1/2, Switch2/3
  Add1/1 -> Switch2/1

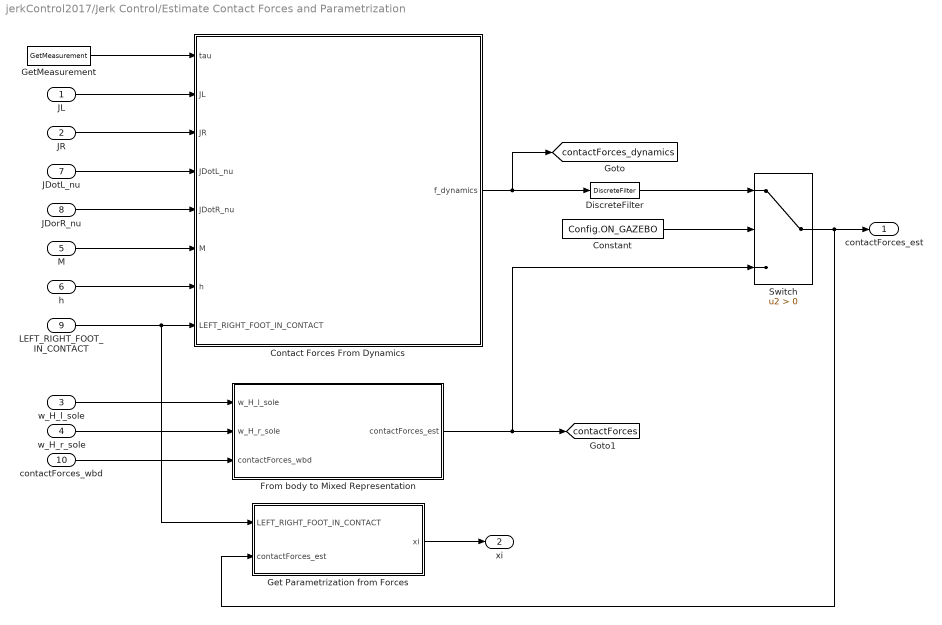
== system jerkControl2017/Jerk Control/Estimate Contact Forces and Parametrization ==
  JL : Inport
  JR : Inport  Port=2
  w_H_l_sole : Inport  Port=3
  w_H_r_sole : Inport  Port=4
  M : Inport  Port=5
  h : Inport  Port=6
  JDotL_nu : Inport  Port=7
  JDorR_nu : Inport  Port=8
  LEFT_RIGHT_FOOT_IN_CONTACT : Inport  Port=9
  contactForces_wbd : Inport  Port=10
  Constant : Constant  Value=Config.ON_GAZEBO
  Contact Forces From Dynamics : MATLAB Function  TreatAsAtomicUnit=on
  DiscreteFilter : WBToolboxLibrary/Utilities/DiscreteFilter  filterType=FirstOrderLowPassFilter  numCoeffs=[0]  denCoeffs=[0]  Fc=10  Ts=Config.Ts  orderMedianFilter=0  initStatus=on  y0=[0;0;150;0;0;0;0;0;150;0;0;0]  u0=[0]
      settings: SourceProductName=WholeBodyToolbox
  From body to Mixed Representation : Subsystem
  Get Parametrization from Forces : Subsystem
  GetMeasurement : WBToolboxLibrary/States/GetMeasurement  measuredType=Joints Torque
      settings: SourceProductName=WholeBodyToolbox
  Switch : Switch  Criteria=u2 > Threshold
  contactForces_est : Outport
  xi : Outport  Port=2
  tag scope: contactForces=global, contactForces_dynamics=global
  wires:
  JDorR_nu/1 -> Contact Forces From Dynamics/5(JDotR_nu)
  JR/1 -> Contact Forces From Dynamics/3(JR)
  JDotL_nu/1 -> Contact Forces From Dynamics/4(JDotL_nu)
  LEFT_RIGHT_FOOT_IN_CONTACT/1 -> Get Parametrization from Forces/1(LEFT_RIGHT_FOOT_IN_CONTACT), Contact Forces From Dynamics/8(LEFT_RIGHT_FOOT_IN_CONTACT)
  h/1 -> Contact Forces From Dynamics/7(h)
  M/1 -> Contact Forces From Dynamics/6(M)
  JL/1 -> Contact Forces From Dynamics/2(JL)
  contactForces_wbd/1 -> From body to Mixed Representation/3(contactForces_wbd)
  w_H_r_sole/1 -> From body to Mixed Representation/2(w_H_r_sole)
  w_H_l_sole/1 -> From body to Mixed Representation/1(w_H_l_sole)
  Switch/1 -> contactForces_est/1, Get Parametrization from Forces/2(contactForces_est)
  From body to Mixed Representation/1(contactForces_est) -> Switch/3, [contactForces]
  Contact Forces From Dynamics/1(f_dynamics) -> DiscreteFilter/1, [contactForces_dynamics]
  GetMeasurement/1 -> Contact Forces From Dynamics/1(tau)
  DiscreteFilter/1 -> Switch/1
  Get Parametrization from Forces/1(xi) -> xi/1
  Constant/1 -> Switch/2

== system jerkControl2017/Jerk Control/Integrate the Input Contact Forces Param. Derivative ==
  xiDot_star : Inport
  LEFT_RIGHT_FOOT_IN_CONTACT : Inport  Port=2
  M : Inport  Port=3
  Demux xiDot : Subsystem
  Discrete-Time Integrator3 : DiscreteIntegrator  ExternalReset=rising  InitialConditionSource=external  InitialConditionSetting=State (most efficient)  SampleTime=Config.Ts  ICPrevOutput=DiscIntNeverNeededParam  ICPrevScaledInput=DiscIntNeverNeededParam
  Discrete-Time Integrator4 : DiscreteIntegrator  ExternalReset=rising  InitialConditionSource=external  InitialConditionSetting=State (most efficient)  SampleTime=Config.Ts  ICPrevOutput=DiscIntNeverNeededParam  ICPrevScaledInput=DiscIntNeverNeededParam
  From Parametrization to Forces : Subsystem
  MatrixMultiply1 : Product
  MatrixMultiply2 : Product
  Mux : Mux  Inputs=2
  Mux1 : Mux  Inputs=2
  deadZone : Subsystem
  xi_star : Outport
  contactForces_star : Outport  Port=2
  tag scope: contactForces_star=global, xiDot_star=global, xi_LFoot_star=global, xi_RFoot_star=global
  wires:
  xiDot_star/1 -> [xiDot_star], deadZone/1(u)
  Demux xiDot/4(xiDot_RFoot) -> Discrete-Time Integrator4/1
  Demux xiDot/5(RFootContactActivation) -> MatrixMultiply2/2, From Parametrization to Forces/4(RFootContactActivation), Discrete-Time Integrator4/2
  Demux xiDot/1(xiDot_LFoot) -> Discrete-Time Integrator3/1
  Mux/1 -> [contactForces_star], contactForces_star/1
  Demux xiDot/2(LFootContactActivation) -> MatrixMultiply1/1, From Parametrization to Forces/1(LFootContactActivation), Discrete-Time Integrator3/2
  deadZone/1(u_cut) -> Demux xiDot/1(xiDot_star)
  LEFT_RIGHT_FOOT_IN_CONTACT/1 -> Demux xiDot/2(LEFT_RIGHT_FOOT_IN_CONTACT)
  M/1 -> Demux xiDot/3(M)
  Demux xiDot/6(init_xi_RFoot) -> Discrete-Time Integrator4/3
  Demux xiDot/3(init_xi_LFoot) -> Discrete-Time Integrator3/3
  Discrete-Time Integrator3/1 -> MatrixMultiply1/2, From Parametrization to Forces/2(xi_LFoot)
  Discrete-Time Integrator4/1 -> From Parametrization to Forces/3(xi_RFoot), MatrixMultiply2/1
  MatrixMultiply1/1 -> Mux1/1, [xi_LFoot_star]
  From Parametrization to Forces/1(contactForces_LFoot) -> Mux/1
  From Parametrization to Forces/2(contactForces_RFoot) -> Mux/2
  MatrixMultiply2/1 -> Mux1/2, [xi_RFoot_star]
  Mux1/1 -> xi_star/1

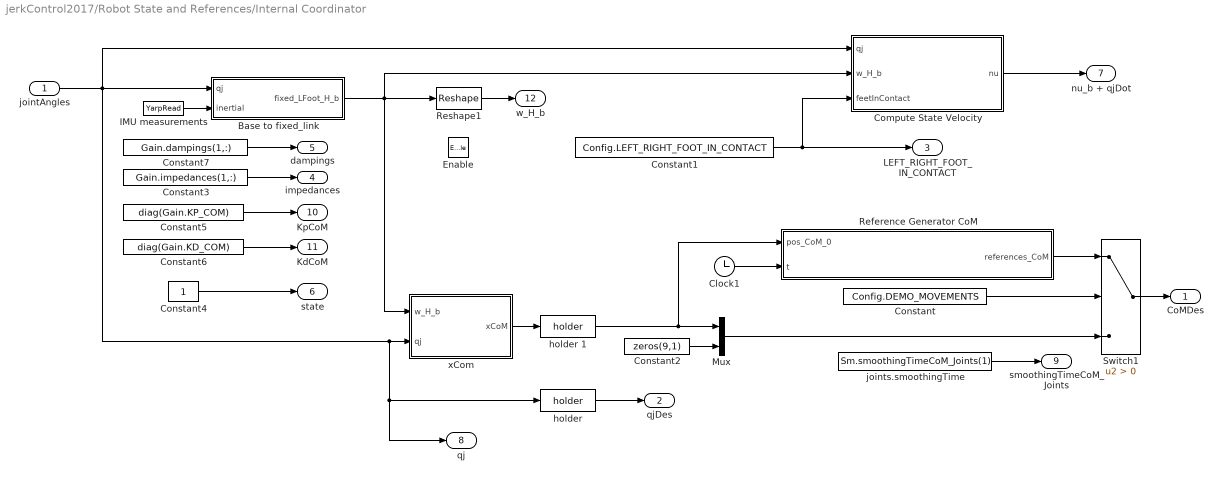
== system jerkControl2017/Robot State and References/Internal Coordinator ==
  jointAngles : Inport
  Enable : EnablePort
  Base to fixed_link : Subsystem
  Clock1 : Clock
  Compute State Velocity : Subsystem
  Constant : Constant  Value=Config.DEMO_MOVEMENTS
  Constant1 : Constant  Value=Config.LEFT_RIGHT_FOOT_IN_CONTACT
  Constant2 : Constant  Value=zeros(9,1)
  Constant3 : Constant  Value=Gain.impedances(1,:)
  Constant4 : Constant
  Constant5 : Constant  Value=diag(Gain.KP_COM)
  Constant6 : Constant  Value=diag(Gain.KD_COM)
  Constant7 : Constant  Value=Gain.dampings(1,:)
  IMU measurements : WBToolboxLibrary/Utilities/YarpRead  portName=Ports.IMU  signalSize=12  timeout=0.5  blocking=off  timestamp=off  autoconnect=on  errorOnConnection=on
      settings: SourceProductName=WholeBodyToolbox
  Mux : Mux  Inputs=2
  Reference Generator CoM : MATLAB Function  TreatAsAtomicUnit=on
  Reshape1 : Reshape  OutputDimensions=[4;4]
  Switch1 : Switch  Criteria=u2 > Threshold
  "holder " : WBToolboxLibrary/Utilities/holder 
      settings: SourceProductName=WholeBodyToolbox
  holder 1 : WBToolboxLibrary/Utilities/holder 
      settings: SourceProductName=WholeBodyToolbox
  joints.smoothingTime : Constant  Value=Sm.smoothingTimeCoM_Joints(1)
  xCom : Subsystem
  CoMDes : Outport
  qjDes : Outport  Port=2
  LEFT_RIGHT_FOOT_IN_CONTACT : Outport  Port=3
  impedances : Outport  Port=4
  dampings : Outport  Port=5
  state : Outport  Port=6
  nu_b + qjDot : Outport  Port=7
  qj : Outport  Port=8
  smoothingTimeCoM_Joints : Outport  Port=9
  KpCoM : Outport  Port=10
  KdCoM : Outport  Port=11
  w_H_b : Outport  Port=12
  wires:
  Constant/1 -> Switch1/2
  "holder "/1 -> qjDes/1
  Switch1/1 -> CoMDes/1
  Mux/1 -> Switch1/3
  Constant2/1 -> Mux/2
  Constant3/1 -> impedances/1
  Constant4/1 -> state/1
  Compute State Velocity/1(nu) -> nu_b + qjDot/1
  holder 1/1 -> Reference Generator CoM/1(pos_CoM_0), Mux/1
  xCom/1(xCoM) -> holder 1/1
  joints.smoothingTime/1 -> smoothingTimeCoM_Joints/1
  jointAngles/1 -> Compute State Velocity/1(qj), Base to fixed_link/1(qj), qj/1, "holder "/1, xCom/2(qj)
  Constant5/1 -> KpCoM/1
  Constant6/1 -> KdCoM/1
  Reshape1/1 -> w_H_b/1
  Constant1/1 -> Compute State Velocity/3("feetInContact "), LEFT_RIGHT_FOOT_IN_CONTACT/1
  IMU measurements/1 -> Base to fixed_link/2(inertial)
  Clock1/1 -> Reference Generator CoM/2(t)
  Reference Generator CoM/1(references_CoM) -> Switch1/1
  Base to fixed_link/1(fixed_LFoot_H_b) -> Compute State Velocity/2(w_H_b), xCom/1(w_H_b), Reshape1/1
  Constant7/1 -> dampings/1

== system jerkControl2017/Robot State and References/Select State and References ==
  StateAndReferences : Inport
  Compute CoM and Joint References : Subsystem
  Demux : Demux  Outputs=[12,ROBOT_DOF,2,ROBOT_DOF,ROBOT_DOF,1,ROBOT_DOF+6,ROBOT_DOF,1,3,3,16]
  Reshape1 : Reshape  OutputDimensionality=Customize  OutputDimensions=[4;4]
  impedances : Outport
  gainsPCOM : Outport  Port=2
  gainsDCOM : Outport  Port=3
  w_H_b : Outport  Port=4
  qj : Outport  Port=5
  nu : Outport  Port=6
  LEFT_RIGHT_FOOT_IN_CONTACT : Outport  Port=7
  desired_x_dx_ddx_dddx_CoM : Outport  Port=8
  qj_dqj_ddqj_des : Outport  Port=9
  state : Outport  Port=10
  dampings : Outport  Port=11
  tag scope: constraints=global, impedances=global, nu=global, smoothingTimes=global
  wires:
  Demux/8 -> qj/1  "qj"
  Demux/6 -> state/1  "state"
  Demux/9 -> [smoothingTimes], Compute CoM and Joint References/3(smoothingTimeMinJerk_CoMDes_qjDes)  "smoothingTimeMinJerk_CoMDes_qjDes"
  Demux/7 -> nu/1, [nu]  "nu"
  StateAndReferences/1 -> Demux/1
  Demux/4 -> [impedances], impedances/1  "impedances"
  Demux/3 -> [constraints], LEFT_RIGHT_FOOT_IN_CONTACT/1  "constraints"
  Reshape1/1 -> w_H_b/1
  Demux/1 -> Compute CoM and Joint References/1(CoMDes)  "CoMDes"
  Demux/2 -> Compute CoM and Joint References/2(qjDes)  "qjDes"
  Compute CoM and Joint References/1(x_dx_ddx_dddx_CoM_des) -> desired_x_dx_ddx_dddx_CoM/1
  Compute CoM and Joint References/2(qj_dqj_ddqj_des) -> qj_dqj_ddqj_des/1
  Demux/12 -> Reshape1/1
  Demux/11 -> gainsDCOM/1
  Demux/10 -> gainsPCOM/1
  Demux/5 -> dampings/1  "dampings"

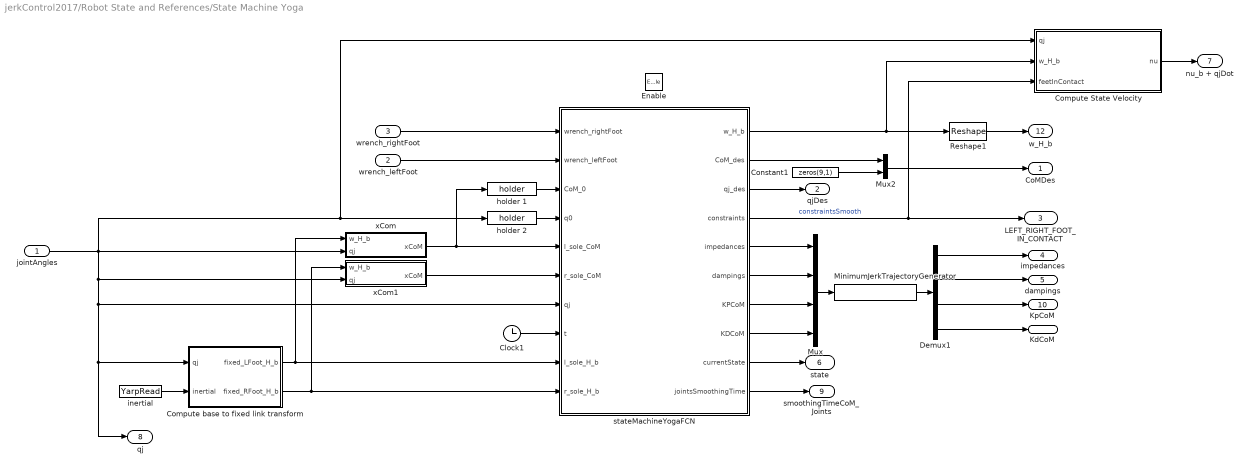
== system jerkControl2017/Robot State and References/State Machine Yoga ==
  jointAngles : Inport
  wrench_leftFoot : Inport  Port=2
  wrench_rightFoot : Inport  Port=3
  Enable : EnablePort
  Clock1 : Clock
  Compute State Velocity : Subsystem
  Compute base to fixed link transform : Subsystem
  Constant1 : Constant  Value=zeros(9,1)
  Demux1 : Demux  Outputs=[ROBOT_DOF,ROBOT_DOF,3,3]
  MinimumJerkTrajectoryGenerator : WBToolboxLibrary/Utilities/MinimumJerkTrajectoryGenerator  externalSettlingTime=off  settlingTime=Gain.SmoothingTimeGainScheduling  sampleTime=Config.Ts  resetOnSettlingTime=off  firstDerivatives=off  secondDerivatives=off  explicitInitialValue=off
      settings: SourceProductName=WholeBodyToolbox
  Mux : Mux
  Mux2 : Mux  Inputs=2
  Reshape1 : Reshape  OutputDimensions=[4;4]
  holder 1 : WBToolboxLibrary/Utilities/holder 
      settings: SourceProductName=WholeBodyToolbox
  holder 2 : WBToolboxLibrary/Utilities/holder 
      settings: SourceProductName=WholeBodyToolbox
  inertial : WBToolboxLibrary/Utilities/YarpRead  portName=Ports.IMU  signalSize=12  timeout=0.5  blocking=off  timestamp=off  autoconnect=on  errorOnConnection=off
      settings: SourceProductName=WholeBodyToolbox
  stateMachineYogaFCN : MATLAB Function  TreatAsAtomicUnit=on
  xCom : Subsystem
  xCom1 : Subsystem
  CoMDes : Outport
  qjDes : Outport  Port=2
  LEFT_RIGHT_FOOT_IN_CONTACT : Outport  Port=3
  impedances : Outport  Port=4
  dampings : Outport  Port=5
  state : Outport  Port=6
  nu_b + qjDot : Outport  Port=7
  qj : Outport  Port=8
  smoothingTimeCoM_Joints : Outport  Port=9
  KpCoM : Outport  Port=10
  KdCoM : Outport  Port=11
  w_H_b : Outport  Port=12
  wires:
  xCom/1(xCoM) -> holder 1/1, stateMachineYogaFCN/5(l_sole_CoM)
  holder 1/1 -> stateMachineYogaFCN/3(CoM_0)
  holder 2/1 -> stateMachineYogaFCN/4(q0)
  Clock1/1 -> stateMachineYogaFCN/8(t)
  stateMachineYogaFCN/3(qj_des) -> qjDes/1
  stateMachineYogaFCN/2(CoM_des) -> Mux2/1
  Mux2/1 -> CoMDes/1
  Constant1/1 -> Mux2/2
  stateMachineYogaFCN/9(currentState) -> state/1
  stateMachineYogaFCN/1(w_H_b) -> Compute State Velocity/2(w_H_b), Reshape1/1
  xCom1/1(xCoM) -> stateMachineYogaFCN/6(r_sole_CoM)
  Compute State Velocity/1(nu) -> nu_b + qjDot/1
  stateMachineYogaFCN/10(jointsSmoothingTime) -> smoothingTimeCoM_Joints/1
  stateMachineYogaFCN/7(KPCoM) -> Mux/3
  Demux1/4 -> KdCoM/1
  stateMachineYogaFCN/8(KDCoM) -> Mux/4
  stateMachineYogaFCN/5(impedances) -> Mux/1
  Mux/1 -> MinimumJerkTrajectoryGenerator/1
  MinimumJerkTrajectoryGenerator/1 -> Demux1/1
  Demux1/1 -> impedances/1
  Demux1/3 -> KpCoM/1
  jointAngles/1 -> xCom/2(qj), Compute State Velocity/1(qj), holder 2/1, qj/1, Compute base to fixed link transform/1(qj), stateMachineYogaFCN/7(qj), xCom1/2(qj)
  Compute base to fixed link transform/1(fixed_LFoot_H_b) -> stateMachineYogaFCN/9(l_sole_H_b), xCom/1(w_H_b)
  Compute base to fixed link transform/2(fixed_RFoot_H_b) -> stateMachineYogaFCN/10(r_sole_H_b), xCom1/1(w_H_b)
  inertial/1 -> Compute base to fixed link transform/2(inertial)
  Reshape1/1 -> w_H_b/1
  wrench_leftFoot/1 -> stateMachineYogaFCN/2(wrench_leftFoot)
  wrench_rightFoot/1 -> stateMachineYogaFCN/1(wrench_rightFoot)
  stateMachineYogaFCN/4(constraints) -> LEFT_RIGHT_FOOT_IN_CONTACT/1, Compute State Velocity/3("feetInContact ")  "constraintsSmooth"
  stateMachineYogaFCN/6(dampings) -> Mux/2
  Demux1/2 -> dampings/1

== system jerkControl2017/emergency stop: joint limits/STOP IF JOINTS HIT THE LIMITS ==
  qj : Inport
  Enable : EnablePort
  Assertion : Assertion
  GetLimits : WBToolboxLibrary/States/GetLimits  limitsSource=ControlBoard  limitsType=Position
      settings: SourceProductName=WholeBodyToolbox
  MATLAB Function : MATLAB Function  TreatAsAtomicUnit=on
  index1 : Constant  Value=0.01  VectorParams1D=off
  wires:
  qj/1 -> MATLAB Function/3(u)
  MATLAB Function/1(inRange) -> Assertion/1
  GetLimits/1 -> MATLAB Function/1(umin)
  GetLimits/2 -> MATLAB Function/2(umax)
  index1/1 -> MATLAB Function/4(tol)
